simulink model "Uby_lqi"  (R2025b)
settings: Solver=VariableStepAuto  StartTime=0.0  StopTime=10.0  RelTol=1e-3
undefined symbols (not defined in the file): A, B, C, D, h0, k_lqi, nx
settings Model: Creator=Miche  LastModifiedBy=Miche

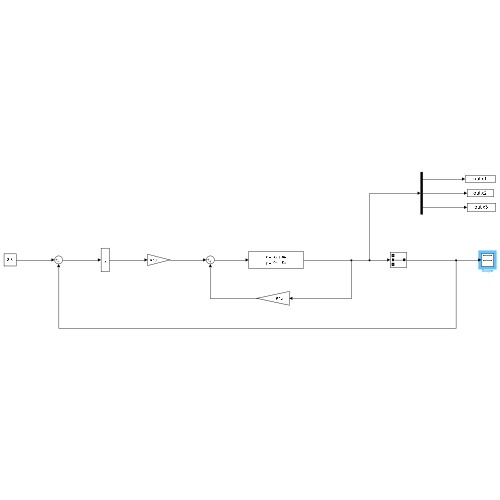
[thumbnail: Simulink's stored preview of the top-level diagram]
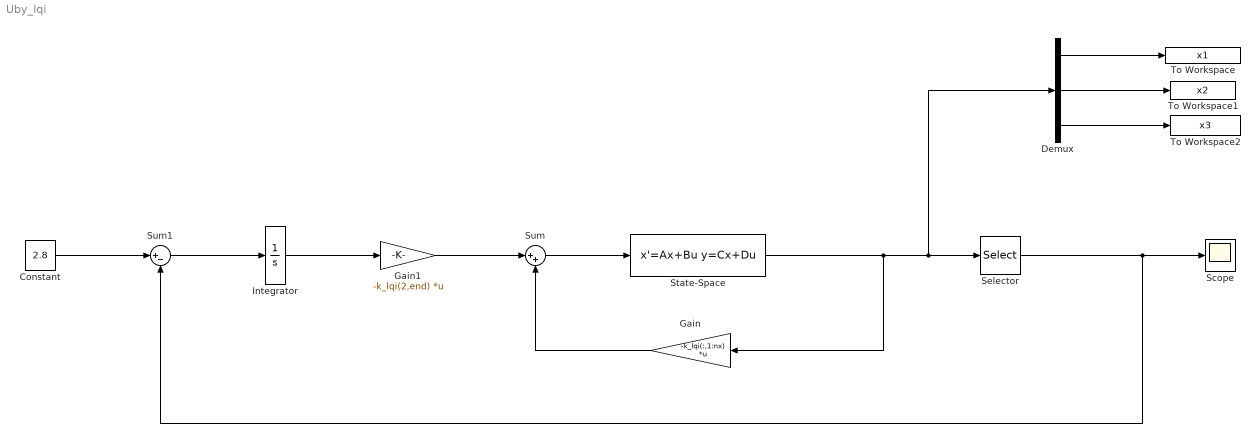
== system Uby_lqi ==
  Constant : Constant  Value=2.8
  Demux : Demux  Outputs=3
  Gain : Gain  Gain=-k_lqi(:,1:nx)  Multiplication=Matrix(K*u)
  Gain1 : Gain  Gain=-k_lqi(2,end)  Multiplication=Matrix(K*u)
  Integrator : Integrator
  Scope : Scope
      settings: ActiveDisplayYMinimum=-0.13675496623639094  ActiveDisplayYMaximum=3.1282724046031989
  Selector : Selector  InputPortWidth=3  IndexOptions=Index vector (dialog)  Indices=2  OutputSizes=1
  State-Space : StateSpace  A=A  B=B  C=C  D=D  InitialCondition=h0
  Sum : Sum  Inputs=|++
  Sum1 : Sum  Inputs=|+-
  To Workspace : ToWorkspace  VariableName=x1  SaveFormat=Timeseries  SampleTime=-1
  To Workspace1 : ToWorkspace  VariableName=x2  SaveFormat=Timeseries  SampleTime=-1
  To Workspace2 : ToWorkspace  VariableName=x3  SaveFormat=Timeseries  SampleTime=-1
  wires:
  Sum/1 -> State-Space/1
  Gain/1 -> Sum/2
  Gain1/1 -> Sum/1
  Integrator/1 -> Gain1/1
  Selector/1 -> Sum1/2, Scope/1
  Sum1/1 -> Integrator/1
  Constant/1 -> Sum1/1
  Demux/1 -> To Workspace/1
  Demux/3 -> To Workspace2/1
  Demux/2 -> To Workspace1/1
  State-Space/1 -> Gain/1, Demux/1, Selector/1
